simulink model "RLC_Simulation"  (R2025b)
settings: Solver=ode23t  StartTime=0.0  StopTime=Sim.t_end  RelTol=1e-3
undefined symbols (not defined in the file): RLC, Sim
libraries: ee_lib x4, fl_lib x2, nesl_utility x2
settings Model: Creator=lucas  LastModifiedBy=marcu
settings DataIOCC: SaveOutput=off  DSMLogging=off  SaveTime=off  ReturnWorkspaceOutputs=off  SignalLoggingName=RLC_SIM

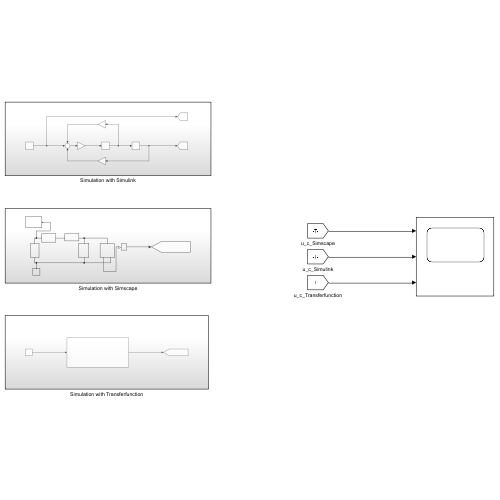
[thumbnail: Simulink's stored preview of the top-level diagram]
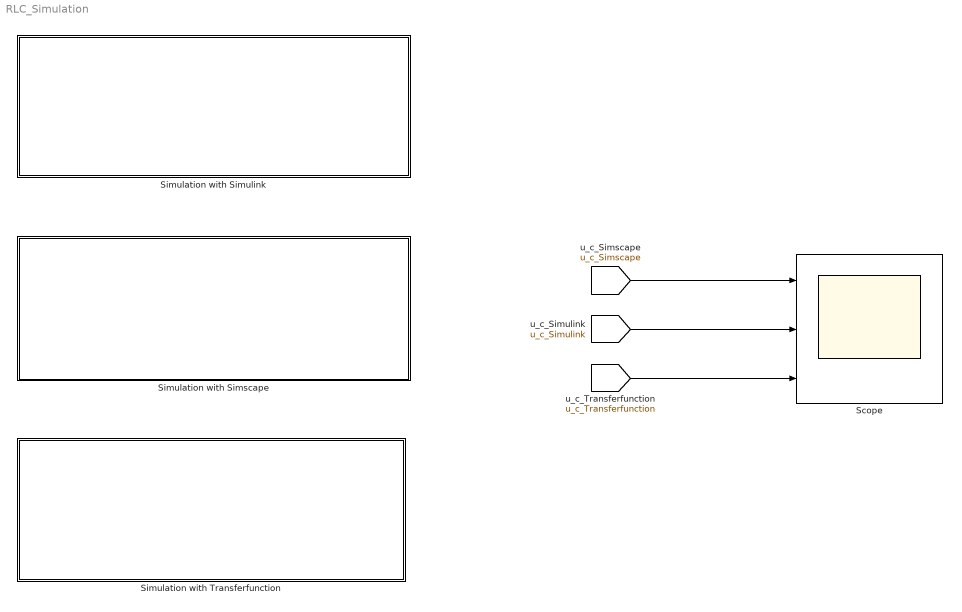
== system RLC_Simulation ==
  Scope : Scope  NumInputPorts=3
      settings: ActiveDisplayYMinimum=-1  ActiveDisplayYMaximum=1
  Simulation with Simscape : Subsystem
  Simulation with Simulink : Subsystem
  Simulation with Transferfunction : Subsystem
  wires:
  [u_c_Simulink] -> Scope/2
  [u_c_Simscape] -> Scope/1
  [u_c_Transferfunction] -> Scope/3

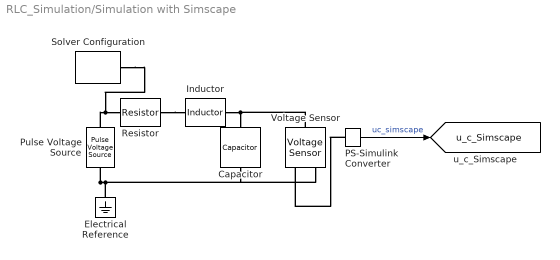
== system RLC_Simulation/Simulation with Simscape ==
  Capacitor : ee_lib/Passive/Capacitor  cap_option=ee.enum.passive.capacitor.capOption.const  c=RLC.C F  Cvec=[1e-05, 1e-06] F  Vvec=[0, 10] V  CV_table_symmetry=ee.enum.passive.capacitor.tableSymmetry.yes  f_vec=[1, 10] kHz  DFext_vec=[.8, 1.2]  enable_C_tol=ee.enum.toleranceApplication.none  averaging_period=0 s  C_tol=5  tol_distribution=ee.enum.toleranceDistribution.uniform  nSigma=4  r=0 Ohm  g=0 1/Ohm  enable_operating_limits=ee.enum.enable.no  operating_limit_action=ee.enum.passive.reportOpLim.warn  max_working_voltage_range=[-25, 25] V  power_rating=1 W  maxTemperature=85 degC  thermalEnable=false  thermalMass=1 J/K  i_specify=off  i_priority=None  i=0 A  i_nominal_specify=off  i_nominal_value=1  i_nominal_unit=A  v_specify=off  v_priority=None  v=0 V  v_nominal_specify=off  v_nominal_value=1  v_nominal_unit=V  vc_specify=off  vc_priority=High  vc=0 V  vc_nominal_specify=off  vc_nominal_value=1  vc_nominal_unit=V  T_specify=off  T_priority=None  T=298.15 K  T_nominal_specify=off  T_nominal_value=1  T_nominal_unit=K
  Electrical Reference : fl_lib/Electrical/Electrical Elements/Electrical Reference
  Inductor : ee_lib/Passive/Inductor  l=RLC.L H  enable_L_tol=ee.enum.toleranceApplication.none  L_tol=20  tol_distribution=ee.enum.toleranceDistribution.uniform  nSigma=4  r=0 Ohm  g=1e-9 1/Ohm  enable_operating_limits=ee.enum.enable.no  operating_limit_action=ee.enum.passive.reportOpLim.warn  max_working_current=1 A  power_rating=1 W  i_L_specify=off  i_L_priority=High  i_L=0 A  i_L_nominal_specify=off  i_L_nominal_value=1  i_L_nominal_unit=A
  PS-Simulink Converter : nesl_utility/PS-Simulink Converter  PhysicalDomain=network_engine_domain  SubClassName=ps_output  LeftPortType=input  RightPortType=output  PseudoPeriodic=off  Frequencies=[]  VectorFormat=inherit  Unit=inherit  AffineConversion=off
  Pulse Voltage Source : ee_lib/Additional Components/SPICE Sources/Pulse Voltage Source  V1=0 V  V2=3 V  TD=2 s  TR=1e-9 s  TF=1e-9 s  PW=Inf s  PER=Inf s
      settings: LibrarySourceBlock=ee_lib/Sources/Pulse Voltage Source  InternalSimscapePortConfiguration="{\"Bottom\":[],\"Left\":[{\"id\":\"p\",\"label\":\"\",\"type\":\"foundation.electrical.electrical\"}],\"Right\":[{\"id\":\"n\",\"label\":\"\",\"type\":\"foundation.electrical.electrical\"}],\"Top\":[]}"
  Resistor : ee_lib/Passive/Resistor  R=RLC.R Ohm  enable_R_tol=ee.enum.toleranceApplication.none  R_tol=5  tol_distribution=ee.enum.toleranceDistribution.uniform  nSigma=4  enable_operating_limits=ee.enum.enable.no  operating_limit_action=ee.enum.passive.reportOpLim.warn  power_rating=1 W  max_working_voltage=100 V  noise_mode=ee.enum.sources.noise.Disabled  Tdevice=25 degC  sample_time=1e-3 s  repeatability=ee.enum.ic.repeatability.notRepeatable  user_seed=0  auto_seed=3499211588  power_derating_T1=70 degC  power_derating_T2=155 degC  operating_temperature_range_vec=[-50, 150] degC  alpha=3.93e-3 1/K  Tmeas=25 degC  thermal_mass=100 J/K  temperature_specify=off  temperature_priority=High  temperature=298.15 K  temperature_nominal_specify=off  temperature_nominal_value=1  temperature_nominal_unit=K
  Solver Configuration : nesl_utility/Solver Configuration  PhysicalDomain=network_engine_domain  SubClassName=solver  LeftPortType=input  RightPortType=generic  Tones=[]  Harmonics=[]  SimulateNoise=off  Profile=off  UseLocalSampling=off  EnableSwitchedLinearOptims=on  FrequencyDomain=off  UseCCode=off  RelTol=0.001  AbsTol=0.001  MinStep=1e-09  ToWorkspace=off  RevertToSquareIcSolve=off  NumHomotopyIterations=100  PhasorMode=off  PhasorModeNumHarmonics=1  ConsistencySolver=NEWTON_XTOL_AFTER_FTOL  IndexReductionMethod=DerivativeReplacement  DoDC=off  ResidualTolerance=1e-09  ConsistencyTolSource=GLOBAL  ConsistencyAbsTol=0.001  ConsistencyRelTol=0.001  ConsistencyTolFactor=0.001  UseLocalSolver=off  LocalSolverChoice=NE_BACKWARD_EULER_ADVANCER  ResolveIndetEquations=on  FunctionEvalNumThread=1  LocalSolverSampleTime=0.001  DoFixedCost=off  MaxNonlinIter=3  MaxModeIter=2  ComputeImpulses=off  ImpulseIterations=2  LinearAlgebra=auto  LinearAlgebraNumThread=0  EquationFormulation=NE_TIME_EF  DelaysMemoryBudget=1024  AutomaticFiltering=on  FilteringTimeConstant=0.001  PartitionStorageMethod=AS_NEEDED  PartitionMemoryBudget=1024  PartitionMethod=ROBUST  MultibodyUseLocalSolver=off  MultibodyLocalSolverChoice=ODE1  MultibodyLocalSolverSampleTime=0.001
  Voltage Sensor : fl_lib/Electrical/Electrical Sensors/Voltage Sensor
  tag scope: u_c_Simscape=global
  wires:
  PS-Simulink Converter/1 -> [u_c_Simscape]  "uc_simscape"
  connections:
  Capacitor/LConn1 -- Inductor/RConn1 -- Voltage Sensor/LConn1
  Pulse Voltage Source/RConn1 -- Capacitor/RConn1 -- Voltage Sensor/RConn2 -- Electrical Reference/LConn1
  PS-Simulink Converter/LConn1 -- Voltage Sensor/RConn1
  Resistor/RConn1 -- Inductor/LConn1
  Resistor/LConn1 -- Pulse Voltage Source/LConn1 -- Solver Configuration/RConn1

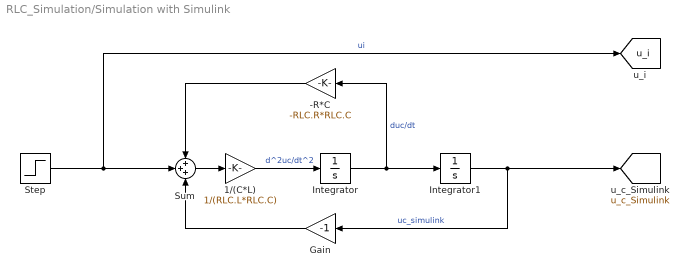
== system RLC_Simulation/Simulation with Simulink ==
  -R*C : Gain  Gain=-RLC.R*RLC.C
  1/(C*L) : Gain  Gain=1/(RLC.L*RLC.C)
  Gain : Gain  Gain=-1
  Integrator : Integrator
  Integrator1 : Integrator
  Step : Step  Time=Sim.t_step  After=RLC.u_i  SampleTime=0
  Sum : Sum  Inputs=+++
  tag scope: u_c_Simulink=global, u_i=global
  wires:
  Integrator1/1 -> [u_c_Simulink], Gain/1  "uc_simulink"
  Integrator/1 -> Integrator1/1, -R*C/1  "duc/dt"
  -R*C/1 -> Sum/1
  Step/1 -> [u_i], Sum/2  "ui"
  1/(C*L)/1 -> Integrator/1  "d^2uc/dt^2"
  Sum/1 -> 1/(C*L)/1
  Gain/1 -> Sum/3

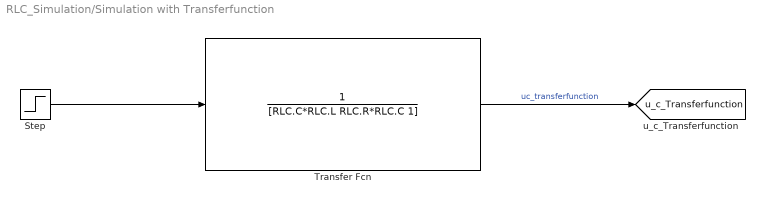
== system RLC_Simulation/Simulation with Transferfunction ==
  Step : Step  Time=Sim.t_step  After=RLC.u_i  SampleTime=0
  Transfer Fcn : TransferFcn  Denominator=[RLC.C*RLC.L RLC.R*RLC.C 1]
  tag scope: u_c_Transferfunction=global
  wires:
  Step/1 -> Transfer Fcn/1
  Transfer Fcn/1 -> [u_c_Transferfunction]  "uc_transferfunction"
